simulink library "fixpt3p1_basic"  (Simulink 6.0)
settings: Solver=ode45  SolverMode=SingleTasking  StartTime=0.0  StopTime=10.0  RelTol=1e-3
undefined symbols (not defined in the file or in its folder): Bias1, Bias2, NumBits1, NumBits2, Slope1, Slope2
libraries: simulink x46, fixpt3p1_basic x2, fixpt_lib_4 x1
settings Model: CovMetricSettings=d  Creator=andyb  LastModifiedBy=andyb  ExtModeAutoUpdateStatusClock=off

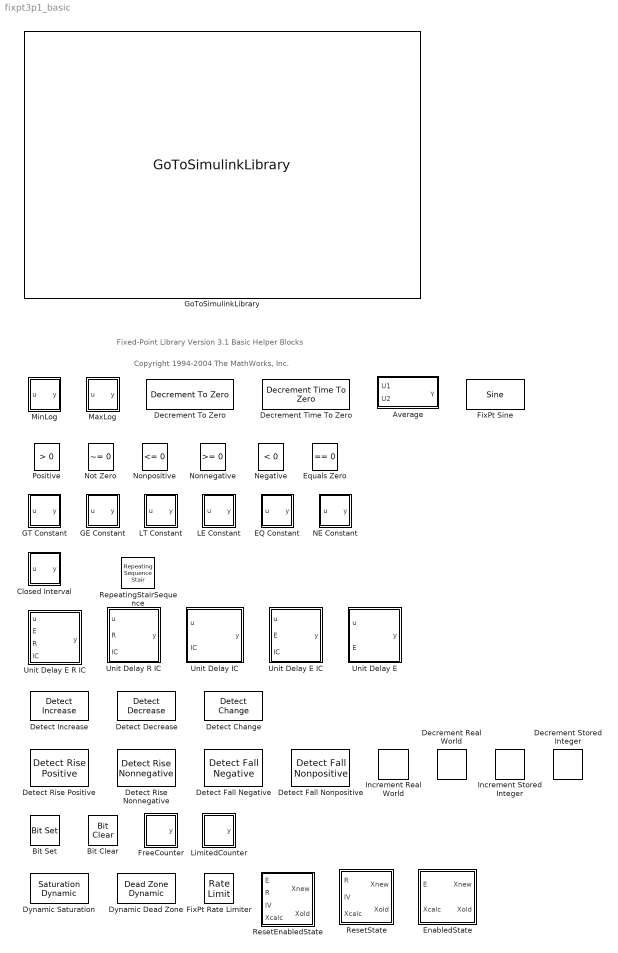
== system fixpt3p1_basic ==
  note: Fixed-Point Library Version 3.1
      | Basic Helper Blocks
  note: Copyright 1994-2004 The MathWorks, Inc.
  Average : Subsystem  PropExecContextAcrossSSBoundary=on
      mask Type: Fixed-Point Average
      mask Description: Compute the average of the two inputs.
      mask Help: fpbhelp('average');
      mask Display:
      | fprintf('(u1+u2) / 2')
      | patch([2 2 10 10 4 4 8 8 4 4 2 ],[2 10 10 8 8 6 6 4 4 2 2 ],[0 0 0],'bottom-right');
  Bit Clear : simulink/Logic and Bit Operations/Bit Clear  iBit=0
  Bit Set : simulink/Logic and Bit Operations/Bit Set  iBit=0
  Closed Interval : Subsystem  PropExecContextAcrossSSBoundary=on  mask(Fixed-Point Closed Interval){uplimit=4, lowlimit=2}
      mask prompts: uplimit "Upper limit:"; lowlimit "Lower Limit:"
      mask help: If the input is in the closed interval between the lower limit and the upper limit, then the output is TRUE, otherwise it is FALSE.
      mask Display:
      | plot([0 1],[0.3 0.3],[0.3 0.3],[0 1],[0 0.2 0.2 0.55 0.55 1],[0.35 0.35 0.6 0.6 0.35 0.35]);
      | patch([2 2 10 10 4 4 8 8 4 4 2 ],[2 10 10 8 8 6 6 4 4 2 2 ],[0 0 0],'bottom-right');
  Decrement Real World : simulink/Additional Math & Discrete/Additional Math: Increment - Decrement/Decrement Real World
  Decrement Stored Integer : simulink/Additional Math & Discrete/Additional Math: Increment - Decrement/Decrement Stored Integer
  Decrement To Zero : simulink/Additional Math & Discrete/Additional Math: Increment - Decrement/Decrement To Zero
  Decrement Time To Zero : simulink/Additional Math & Discrete/Additional Math: Increment - Decrement/Decrement Time To Zero
  Detect Change : simulink/Logic and Bit Operations/Detect Change  vinit=0
  Detect Decrease : simulink/Logic and Bit Operations/Detect Decrease  vinit=0.0
  Detect Increase : simulink/Logic and Bit Operations/Detect Increase  vinit=0.0
  Detect Fall Negative : simulink/Logic and Bit Operations/Detect Fall Negative  vinit=0
  Detect Fall Nonpositive : simulink/Logic and Bit Operations/Detect Fall Nonpositive  vinit=0
  Detect Rise Nonnegative : simulink/Logic and Bit Operations/Detect Rise Nonnegative  vinit=0
  Detect Rise Positive : simulink/Logic and Bit Operations/Detect Rise Positive  vinit=0
  Dynamic Dead Zone : simulink/Discontinuities/Dead Zone Dynamic
  Dynamic Saturation : simulink/Discontinuities/Saturation Dynamic
  EQ Constant : Subsystem  PropExecContextAcrossSSBoundary=on  mask(Fixed-Point Equal To Constant){const=3.0}
      mask prompts: const "Constant value:"
      mask help: Determine if a signal is equal to a constant.
      mask init:
      | if length(const) == 1
      |  str = ['== ',num2str(const)];
      | else
      |   str = '== C';
      | end
      mask Help: fpbhelp('eqconstant');
      mask CallbackString: fixptdialog(gcbh)
      mask Display:
      | disp(str)
      | patch([2 2 10 10 4 4 8 8 4 4 2 ],[2 10 10 8 8 6 6 4 4 2 2 ],[0 0 0],'bottom-right');
  EnabledState : Subsystem  PropExecContextAcrossSSBoundary=on
      mask Type: Fixed-Point Reset Enabled State
      mask Description:
      | Resetable Enabled State
      | Start
      |   Xold = 0.0
      | Output
      |   If E % Enabled
      |      Xnew = Xcalc
      |   else
      |      Xnew = Xold % Stays the same
      |   end
      | Update
      |     Xold = Xnew
      mask Help: fpbhelp('enabledstate');
      mask Display:
      | fprintf('State')
      | patch([2 2 10 10 4 4 8 8 4 4 2 ],[2 10 10 8 8 6 6 4 4 2 2 ],[0 0 0],'bottom-right');
  Equals Zero : simulink/Logic and Bit Operations/Compare To Zero  relop===  LogicOutDataTypeMode=uint8
  FixPt Rate Limiter : RateLimiter  RisingSlewLimit=2  FallingSlewLimit=-2
  FixPt Sine : simulink/Lookup Tables/Sine  NumDataPoints=(2^5)+1
  FreeCounter : Subsystem  PropExecContextAcrossSSBoundary=on  mask(Fixed-Point Free Counter){NumBits=16, tsamp=-1}
      mask prompts: NumBits "Number of Bits"; tsamp "Sample time:"
      mask help:
      | This block is a counter that overflows back to zero after it has reached the maximum value possible for the specified number of bits. The count is always initialized to zero.  The output is normally an unsigned integer.
      |
      | WARNING: This block is intended to overflow.  When global doubles override is on, this block will not wrap back to zero as expected.
      mask Help: fpbhelp('freecounter');
      mask Display:
      | plot( 0.05+0.9/8*[0 1 1 2 2 3 3 4 4 5 5 6 6 7 7 8 8], 0.3+0.65/3*[0 0 1 1 2 2 3 3 0 0 1 1 2 2 3 3 0] )
      | patch([2 2 10 10 4 4 8 8 4 4 2 ],[2 10 10 8 8 6 6 4 4 2 2 ],[0 0 0],'bottom-right');
  GE Constant : Subsystem  PropExecContextAcrossSSBoundary=on  mask(Fixed-Point Greater Than or Equal To Constant){const=3.0}
      mask prompts: const "Constant value:"
      mask help: Determine if a signal is greater than or equal to a constant.
      mask init:
      | if length(const) == 1
      |  str = ['>= ',num2str(const)];
      | else
      |   str = '>= C';
      | end
      mask Help: fpbhelp('geconstant');
      mask CallbackString: fixptdialog(gcbh)
      mask Display:
      | disp(str)
      | patch([2 2 10 10 4 4 8 8 4 4 2 ],[2 10 10 8 8 6 6 4 4 2 2 ],[0 0 0],'bottom-right');
  GT Constant : Subsystem  PropExecContextAcrossSSBoundary=on  mask(Fixed-Point Strictly Greater Than Constant){const=3.0}
      mask prompts: const "Constant value:"
      mask help: Determine if a signal is strictly greater than a constant.
      mask init:
      | if length(const) == 1
      |  str = ['> ',num2str(const)];
      | else
      |   str = '> C';
      | end
      mask Help: fpbhelp('gtconstant');
      mask CallbackString: fixptdialog(gcbh)
      mask Display:
      | disp(str)
      | patch([2 2 10 10 4 4 8 8 4 4 2 ],[2 10 10 8 8 6 6 4 4 2 2 ],[0 0 0],'bottom-right');
  GoToSimulinkLibrary : fixpt_lib_4/GoToSimulinkLibrary
  Increment Real World : simulink/Additional Math & Discrete/Additional Math: Increment - Decrement/Increment Real World
  Increment Stored Integer : simulink/Additional Math & Discrete/Additional Math: Increment - Decrement/Increment Stored Integer
  LE Constant : Subsystem  PropExecContextAcrossSSBoundary=on  mask(Fixed-Point Less Than Or Equal To Constant){const=3.0}
      mask prompts: const "Constant value:"
      mask help: Determine if a signal is less than or equal to a constant.
      mask init:
      | if length(const) == 1
      |  str = ['<= ',num2str(const)];
      | else
      |   str = '<= C';
      | end
      mask Help: fpbhelp('leconstant');
      mask CallbackString: fixptdialog(gcbh)
      mask Display:
      | disp(str)
      | patch([2 2 10 10 4 4 8 8 4 4 2 ],[2 10 10 8 8 6 6 4 4 2 2 ],[0 0 0],'bottom-right');
  LT Constant : Subsystem  PropExecContextAcrossSSBoundary=on  mask(Fixed-Point Strictly Less Than Constant){const=3.0}
      mask prompts: const "Constant value:"
      mask help: Determine if a signal is strictly less than a constant.
      mask init:
      | if length(const) == 1
      |  str = ['< ',num2str(const)];
      | else
      |   str = '< C';
      | end
      mask Help: fpbhelp('ltconstant');
      mask CallbackString: fixptdialog(gcbh)
      mask Display:
      | disp(str)
      | patch([2 2 10 10 4 4 8 8 4 4 2 ],[2 10 10 8 8 6 6 4 4 2 2 ],[0 0 0],'bottom-right');
  LimitedCounter : Subsystem  PropExecContextAcrossSSBoundary=on  mask(Fixed-Point Limited Counter){uplimit=7, tsamp=-1}
      mask prompts: uplimit "Upper limit:"; tsamp "Sample time:"
      mask help: This block is a counter that wraps back to zero after it has output the specified upper limit. The count is always initialized to zero. The output is normally an unsigned integer of 8, 16, or 32 bits. The smallest number of bits needed to represent the upper limit is used.
      mask init:
      | upMax = max(uplimit);
      | if upMax <= (2^8-1)
      |   nbits = 8;
      | elseif upMax <= (2^16-1)
      |   nbits = 16;
      | elseif upMax <= (2^32-1)
      |   nbits = 32;
      | elseif upMax <= (2^64-1)
      |   nbits = 64;
      | else
      |   nbits = 128;
      | end
      mask Help: fpbhelp('limitedcounter');
      mask Display:
      | plot( 0.15+0.8/8*[0 1 1 2 2 3 3 4 4 5 5 6 6 7 7 8 8], 0.3+0.65/3*[0 0 1 1 2 2 3 3 0 0 1 1 2 2 3 3 0] )
      | text(0.05,0.85,'lim')
      | patch([2 2 10 10 4 4 8 8 4 4 2 ],[2 10 10 8 8 6 6 4 4 2 2 ],[0 0 0],'bottom-right');
  MaxLog : Subsystem  PropExecContextAcrossSSBoundary=on
      mask Type: Fixed-Point Running Maximum
      mask Description:
      | Output is the maximum value of the input since the simulation began.
      | 
      | The initial value is currently set to zero!!!!!!
      mask Help: fpbhelp('maxlog');
      mask Display:
      | disp('max\nlog')
      | patch([2 2 10 10 4 4 8 8 4 4 2 ],[2 10 10 8 8 6 6 4 4 2 2 ],[0 0 0],'bottom-right');
  MinLog : Subsystem  PropExecContextAcrossSSBoundary=on
      mask Type: Fixed-Point Running Minimum
      mask Description:
      | Output is the minimum value of the input since the simulation began.
      | 
      | The initial value is currently set to zero!!!!!!
      mask Help: fpbhelp('minlog');
      mask Display:
      | disp('min\nlog')
      | patch([2 2 10 10 4 4 8 8 4 4 2 ],[2 10 10 8 8 6 6 4 4 2 2 ],[0 0 0],'bottom-right');
  NE Constant : Subsystem  PropExecContextAcrossSSBoundary=on  mask(Fixed-Point Not Equal To Constant){const=3.0}
      mask prompts: const "Constant value:"
      mask help: Determine if a signal is not equal to a constant.
      mask init:
      | if length(const) == 1
      |  str = ['~= ',num2str(const)];
      | else
      |   str = '~= C';
      | end
      mask Help: fpbhelp('neconstant');
      mask CallbackString: fixptdialog(gcbh)
      mask Display:
      | disp(str)
      | patch([2 2 10 10 4 4 8 8 4 4 2 ],[2 10 10 8 8 6 6 4 4 2 2 ],[0 0 0],'bottom-right');
  Negative : simulink/Logic and Bit Operations/Compare To Zero  relop=<  LogicOutDataTypeMode=uint8
  Nonnegative : simulink/Logic and Bit Operations/Compare To Zero  relop=>=  LogicOutDataTypeMode=uint8
  Nonpositive : simulink/Logic and Bit Operations/Compare To Zero  relop=<=  LogicOutDataTypeMode=uint8
  Not Zero : simulink/Logic and Bit Operations/Compare To Zero  relop=~=  LogicOutDataTypeMode=uint8
  Positive : simulink/Logic and Bit Operations/Compare To Zero  relop=>  LogicOutDataTypeMode=uint8
  RepeatingStairSequence : simulink/Sources/Repeating Sequence Stair  OutValues=[3 1 4 2 1].'  tsamp=-1  OutputDataTypeScalingMode=Specify via dialog  OutDataType=sfix(16)  ConRadixGroup=Best Precision: Vector-wise  OutScaling=2^-10
  ResetEnabledState : Subsystem  PropExecContextAcrossSSBoundary=on
      mask Type: Fixed-Point Reset Enabled State
      mask Description:
      | Resetable Enabled State
      | Start
      |   Xold = 0.0
      | Output
      |   If R % Reset
      |      Xnew = IV
      |   elseif E % Enabled
      |      Xnew = Xcalc
      |   else
      |      Xnew = Xold % Stays the same
      |   end
      | Update
      |     Xold = Xnew
      mask Help: fpbhelp('resetenabledstate');
      mask Display:
      | fprintf('State')
      | patch([2 2 10 10 4 4 8 8 4 4 2 ],[2 10 10 8 8 6 6 4 4 2 2 ],[0 0 0],'bottom-right');
  ResetState : Subsystem  PropExecContextAcrossSSBoundary=on
      mask Type: Fixed-Point Reset State
      mask Description:
      | Resetable State
      | Start
      |   Xold = 0.0
      | Output
      |   If R % Reset
      |      Xnew = IV
      |   else
      |      Xnew = Xcalc
      |   end
      | Update
      |     Xold = Xnew
      mask Help: fpbhelp('resetstate');
      mask Display:
      | fprintf('State')
      | patch([2 2 10 10 4 4 8 8 4 4 2 ],[2 10 10 8 8 6 6 4 4 2 2 ],[0 0 0],'bottom-right');
  Unit Delay E : Subsystem  PropExecContextAcrossSSBoundary=on  mask(Fixed-Point Unit Delay Enable){vinit=0.0, tsamp=-1}
      mask prompts: vinit "Initial condition:"; tsamp "Sample time:"
      mask help:
      | Enabled Unit Delay
      | Start
      |   x = IC   % Initial Condition
      | Output
      |   y = IC   % Initial Condition
      | Update
      |   If E   % Enabled
      |      x = u
      |   else
      |      % x stays the same
      |   end
      mask Help: fpbhelp('unitdelaye');
      mask Display:
      | dpoly(1,[1 0],'z')
      | patch([2 2 10 10 4 4 8 8 4 4 2 ],[2 10 10 8 8 6 6 4 4 2 2 ],[0 0 0],'bottom-right');
  Unit Delay E IC : Subsystem  PropExecContextAcrossSSBoundary=on  mask(Fixed-Point Unit Delay Enable Initial_Condition){tsamp=-1}
      mask prompts: tsamp "Sample time:"
      mask help:
      | Enabled Unit Delay with External Initial Condition
      | Start
      |   x = IC   % Initial Condition
      | Output
      |   y = IC   % Initial Condition
      | Update
      |   If E   % Enabled
      |      x = u
      |   else
      |      % x stays the same
      |   end
      mask Help: fpbhelp('unitdelayeic');
      mask Display:
      | dpoly(1,[1 0],'z')
      | patch([2 2 10 10 4 4 8 8 4 4 2 ],[2 10 10 8 8 6 6 4 4 2 2 ],[0 0 0],'bottom-right');
  Unit Delay E R IC : Subsystem  PropExecContextAcrossSSBoundary=on  mask(Fixed-Point Unit Delay Reset Enable Initial_Condition){tsamp=-1}
      mask prompts: tsamp "Sample time:"
      mask help:
      | Resetable Enabled Unit Delay with External Initial Condition
      | Start
      |   x = IC   % Initial Condition
      | Output
      |   If R   % Reset
      |      y = IC   % Initial Condition
      |   else
      |      y = x
      |   end
      | Update
      |   If R   % Reset
      |      x = IC   % Initial Condition
      |   elseif E   % Enabled
      |      x = u
      |   else
      |      % x stays the same
      |   end
      mask Help: fpbhelp('unitdelayeric');
      mask Display:
      | dpoly(1,[1 0],'z')
      | patch([2 2 10 10 4 4 8 8 4 4 2 ],[2 10 10 8 8 6 6 4 4 2 2 ],[0 0 0],'bottom-right');
  Unit Delay IC : Subsystem  PropExecContextAcrossSSBoundary=on  mask(Fixed-Point Unit Delay Initial_Condition){tsamp=-1}
      mask prompts: tsamp "Sample time:"
      mask help:
      | Unit Delay with External Initial Condition
      | Start
      |   x = IC   % Initial Condition
      | Output
      |   y = x
      | Update
      |   x = u
      mask Help: fpbhelp('unitdelayic');
      mask Display:
      | dpoly(1,[1 0],'z')
      | patch([2 2 10 10 4 4 8 8 4 4 2 ],[2 10 10 8 8 6 6 4 4 2 2 ],[0 0 0],'bottom-right');
  Unit Delay R IC : Subsystem  PropExecContextAcrossSSBoundary=on  mask(Fixed-Point Unit Delay Reset Initial_Condition){tsamp=-1}
      mask prompts: tsamp "Sample time:"
      mask help:
      | Resetable Unit Delay with External Initial Condition
      | Start
      |   x = IC   % Initial Condition
      | Output
      |   If R   % Reset
      |      y = IC   % Initial Condition
      |   else
      |      y = x
      |   end
      | Update
      |   If R   % Reset
      |      x = IC   % Initial Condition
      |   else
      |      x = u
      |   end
      mask Help: fpbhelp('unitdelayric');
      mask Display:
      | dpoly(1,[1 0],'z')
      | patch([2 2 10 10 4 4 8 8 4 4 2 ],[2 10 10 8 8 6 6 4 4 2 2 ],[0 0 0],'bottom-right');

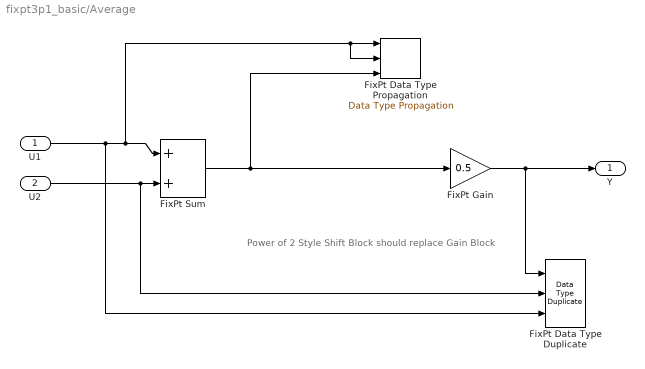
== system fixpt3p1_basic/Average ==
  note: Power of 2 Style Shift Block
      | should replace Gain Block
  U1 : Inport  LatchInput=off
  U2 : Inport  Port=2  LatchInput=off
  FixPt Data Type Duplicate : simulink/Signal Attributes/Data Type Duplicate  NumInputPorts=3
  FixPt Data Type Propagation : simulink/Signal Attributes/Data Type Propagation  PropDataType=sfix(16)  IfRefDouble=double  IfRefSingle=single  IsSigned=IsSigned1  NumBitsBase=NumBits1  NumBitsMult=2  NumBitsAdd=0  NumBitsAllowFinal=1:128  PropScaling=2^-10  ValuesUsedBestPrec=[5 -7]  SlopeBase=Slope1  SlopeMult=1  SlopeAdd=0  BiasBase=Bias1+Bias2  BiasMult=1  BiasAdd=0
  FixPt Gain : Gain  Gain=0.5  ParameterDataTypeMode=Specify via dialog  ParameterDataType=ufix(8)  ParameterScalingMode=Use specified scaling  ParameterScaling=2^-1  OutScaling=2^-10
  FixPt Sum : Sum  OutScaling=2^-10
  Y : Outport  InitialOutput=0
  wires:
  FixPt Gain/1 -> Y/1, FixPt Data Type Duplicate/1
  U1/1 -> FixPt Sum/1, FixPt Data Type Propagation/1, FixPt Data Type Propagation/2, FixPt Data Type Duplicate/3
  U2/1 -> FixPt Sum/2, FixPt Data Type Duplicate/2
  FixPt Sum/1 -> FixPt Gain/1, FixPt Data Type Propagation/3

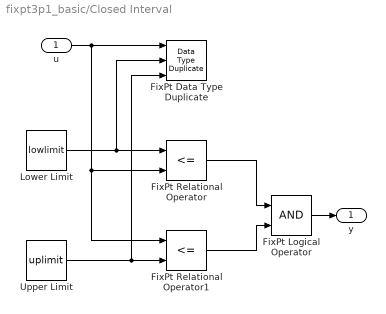
== system fixpt3p1_basic/Closed Interval ==
  u : Inport  LatchInput=off
  FixPt Data Type Duplicate : simulink/Signal Attributes/Data Type Duplicate  NumInputPorts=3
  FixPt Logical Operator : Logic  AllPortsSameDT=off  OutDataTypeMode=Specify via dialog
  FixPt Relational Operator : RelationalOperator  Operator=<=  LogicOutDataTypeMode=Specify via dialog  ZeroCross=off
  FixPt Relational Operator1 : RelationalOperator  Operator=<=  LogicOutDataTypeMode=Specify via dialog  ZeroCross=off
  Lower Limit : Constant  Value=lowlimit  ConRadixGroup=Best Precision: Vector-wise  OutScaling=2^-1000
  Upper Limit : Constant  Value=uplimit  ConRadixGroup=Best Precision: Vector-wise  OutScaling=2^-1000
  y : Outport
  wires:
  Lower Limit/1 -> FixPt Relational Operator/1, FixPt Data Type Duplicate/2
  Upper Limit/1 -> FixPt Relational Operator1/2, FixPt Data Type Duplicate/3
  FixPt Relational Operator/1 -> FixPt Logical Operator/1
  FixPt Relational Operator1/1 -> FixPt Logical Operator/2
  u/1 -> FixPt Data Type Duplicate/1, FixPt Relational Operator/2, FixPt Relational Operator1/1
  FixPt Logical Operator/1 -> y/1

== system fixpt3p1_basic/EQ Constant ==
  u : Inport  LatchInput=off
  FixPt Constant : Constant  Value=const  OutScaling=1
  FixPt Data Type Duplicate : simulink/Signal Attributes/Data Type Duplicate  NumInputPorts=2
  FixPt Relational Operator : RelationalOperator  Operator===  LogicOutDataTypeMode=Specify via dialog  ZeroCross=off
  y : Outport
  wires:
  FixPt Relational Operator/1 -> y/1
  FixPt Constant/1 -> FixPt Data Type Duplicate/2, FixPt Relational Operator/2
  u/1 -> FixPt Data Type Duplicate/1, FixPt Relational Operator/1

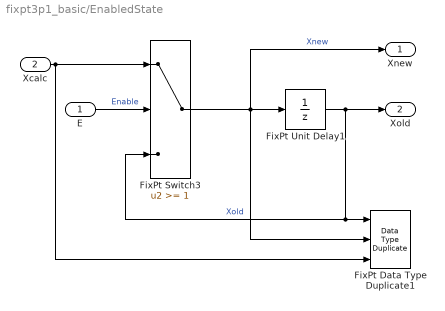
== system fixpt3p1_basic/EnabledState ==
  E : Inport  LatchInput=off
  Xcalc : Inport  Port=2  LatchInput=off
  FixPt Data Type Duplicate1 : simulink/Signal Attributes/Data Type Duplicate  NumInputPorts=3
  FixPt Switch3 : Switch  Threshold=1  ZeroCross=off
  FixPt Unit Delay1 : UnitDelay  X0=0.0  SampleTime=-1
  Xnew : Outport
  Xold : Outport  Port=2
  wires:
  E/1 -> FixPt Switch3/2  "Enable"
  Xcalc/1 -> FixPt Data Type Duplicate1/3, FixPt Switch3/1
  FixPt Switch3/1 -> Xnew/1, FixPt Data Type Duplicate1/2, FixPt Unit Delay1/1  "Xnew"
  FixPt Unit Delay1/1 -> Xold/1, FixPt Switch3/3, FixPt Data Type Duplicate1/1  "Xold"

== system fixpt3p1_basic/FreeCounter ==
  FixPt Data Type Propagation : simulink/Signal Attributes/Data Type Propagation  PropDataTypeMode=Specify via dialog  PropDataType=uint(NumBits)  IfRefDouble=double  IfRefSingle=single  IsSigned=IsSigned1 or IsSigned2  NumBitsBase=max([NumBits1 NumBits2])  NumBitsMult=1  NumBitsAdd=0  NumBitsAllowFinal=1:128  PropScalingMode=Specify via dialog  PropScaling=1  ValuesUsedBestPrec=[5 -7]  SlopeBase=min([Slope1 Slope2])  SlopeMult=1  SlopeAdd=0  BiasBase=Bias1  BiasMult=1  BiasAdd=0
  FixPt Unit Delay2 : UnitDelay  X0=0.0  SampleTime=tsamp
  Increment Real World : fixpt3p1_basic/Increment Real World
  y : Outport
  wires:
  Increment Real World/1 -> FixPt Unit Delay2/1, FixPt Data Type Propagation/1, FixPt Data Type Propagation/3, FixPt Data Type Propagation/2
  FixPt Unit Delay2/1 -> y/1, Increment Real World/1

== system fixpt3p1_basic/GE Constant ==
  u : Inport  LatchInput=off
  FixPt Constant : Constant  Value=const  OutScaling=1
  FixPt Data Type Duplicate : simulink/Signal Attributes/Data Type Duplicate  NumInputPorts=2
  FixPt Relational Operator : RelationalOperator  LogicOutDataTypeMode=Specify via dialog  ZeroCross=off
  y : Outport
  wires:
  u/1 -> FixPt Relational Operator/1, FixPt Data Type Duplicate/1
  FixPt Constant/1 -> FixPt Relational Operator/2, FixPt Data Type Duplicate/2
  FixPt Relational Operator/1 -> y/1

== system fixpt3p1_basic/GT Constant ==
  u : Inport  LatchInput=off
  FixPt Constant : Constant  Value=const  OutScaling=1
  FixPt Data Type Duplicate : simulink/Signal Attributes/Data Type Duplicate  NumInputPorts=2
  FixPt Relational Operator : RelationalOperator  Operator=>  LogicOutDataTypeMode=Specify via dialog  ZeroCross=off
  y : Outport
  wires:
  FixPt Relational Operator/1 -> y/1
  FixPt Constant/1 -> FixPt Data Type Duplicate/2, FixPt Relational Operator/2
  u/1 -> FixPt Data Type Duplicate/1, FixPt Relational Operator/1

== system fixpt3p1_basic/LE Constant ==
  u : Inport  LatchInput=off
  FixPt Constant : Constant  Value=const  OutScaling=1
  FixPt Data Type Duplicate : simulink/Signal Attributes/Data Type Duplicate  NumInputPorts=2
  FixPt Relational Operator : RelationalOperator  Operator=<=  LogicOutDataTypeMode=Specify via dialog  ZeroCross=off
  y : Outport
  wires:
  u/1 -> FixPt Relational Operator/1, FixPt Data Type Duplicate/1
  FixPt Constant/1 -> FixPt Relational Operator/2, FixPt Data Type Duplicate/2
  FixPt Relational Operator/1 -> y/1

== system fixpt3p1_basic/LT Constant ==
  u : Inport  LatchInput=off
  FixPt Constant : Constant  Value=const  OutScaling=1
  FixPt Data Type Duplicate : simulink/Signal Attributes/Data Type Duplicate  NumInputPorts=2
  FixPt Relational Operator : RelationalOperator  Operator=<  LogicOutDataTypeMode=Specify via dialog  ZeroCross=off
  y : Outport
  wires:
  FixPt Relational Operator/1 -> y/1
  FixPt Constant/1 -> FixPt Data Type Duplicate/2, FixPt Relational Operator/2
  u/1 -> FixPt Data Type Duplicate/1, FixPt Relational Operator/1

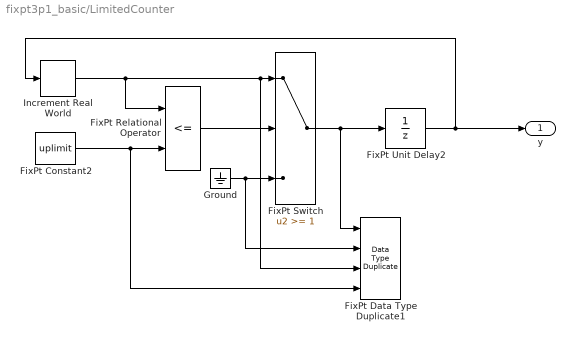
== system fixpt3p1_basic/LimitedCounter ==
  FixPt Constant2 : Constant  Value=uplimit  OutDataTypeMode=Specify via dialog  OutDataType=uint(nbits)  OutScaling=1
  FixPt Data Type Duplicate1 : simulink/Signal Attributes/Data Type Duplicate  NumInputPorts=4
  FixPt Relational Operator : RelationalOperator  Operator=<=  LogicOutDataTypeMode=Specify via dialog  ZeroCross=off
  FixPt Switch : Switch  Threshold=1  ZeroCross=off
  FixPt Unit Delay2 : UnitDelay  X0=0.0  SampleTime=tsamp
  Ground : Ground
  Increment Real World : fixpt3p1_basic/Increment Real World
  y : Outport
  wires:
  FixPt Constant2/1 -> FixPt Data Type Duplicate1/4, FixPt Relational Operator/2
  FixPt Relational Operator/1 -> FixPt Switch/2
  FixPt Unit Delay2/1 -> Increment Real World/1, y/1
  FixPt Switch/1 -> FixPt Unit Delay2/1, FixPt Data Type Duplicate1/1
  Increment Real World/1 -> FixPt Data Type Duplicate1/3, FixPt Switch/1, FixPt Relational Operator/1
  Ground/1 -> FixPt Switch/3, FixPt Data Type Duplicate1/2

== system fixpt3p1_basic/MaxLog ==
  u : Inport  LatchInput=off
  FixPt Data Type Duplicate : simulink/Signal Attributes/Data Type Duplicate  NumInputPorts=3
  FixPt Unit Delay : UnitDelay  X0=0.0  SampleTime=-1
  max low : MinMax  Function=max  Inputs=2  OutScaling=2^-10  ZeroCross=off
  y : Outport
  wires:
  max low/1 -> FixPt Data Type Duplicate/1, FixPt Unit Delay/1
  u/1 -> FixPt Data Type Duplicate/3, max low/1
  FixPt Unit Delay/1 -> FixPt Data Type Duplicate/2, max low/2, y/1

== system fixpt3p1_basic/MinLog ==
  u : Inport  LatchInput=off
  FixPt Data Type Duplicate : simulink/Signal Attributes/Data Type Duplicate  NumInputPorts=3
  FixPt Unit Delay : UnitDelay  X0=0.0  SampleTime=-1
  min : MinMax  Inputs=2  OutScaling=2^-10  ZeroCross=off
  y : Outport
  wires:
  FixPt Unit Delay/1 -> min/2, FixPt Data Type Duplicate/2, y/1
  u/1 -> min/1, FixPt Data Type Duplicate/3
  min/1 -> FixPt Unit Delay/1, FixPt Data Type Duplicate/1

== system fixpt3p1_basic/NE Constant ==
  u : Inport  LatchInput=off
  FixPt Constant : Constant  Value=const  OutScaling=1
  FixPt Data Type Duplicate : simulink/Signal Attributes/Data Type Duplicate  NumInputPorts=2
  FixPt Relational Operator : RelationalOperator  Operator=~=  LogicOutDataTypeMode=Specify via dialog  ZeroCross=off
  y : Outport
  wires:
  u/1 -> FixPt Relational Operator/1, FixPt Data Type Duplicate/1
  FixPt Constant/1 -> FixPt Relational Operator/2, FixPt Data Type Duplicate/2
  FixPt Relational Operator/1 -> y/1

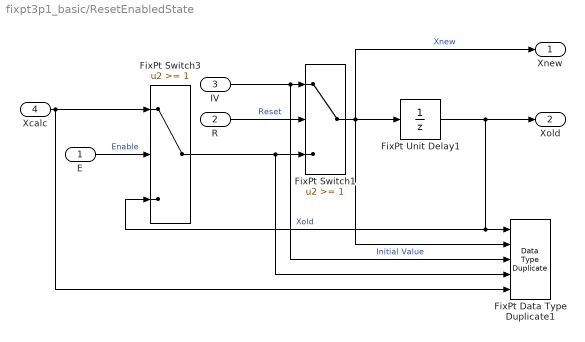
== system fixpt3p1_basic/ResetEnabledState ==
  E : Inport  LatchInput=off
  R : Inport  Port=2  LatchInput=off
  IV : Inport  Port=3  LatchInput=off
  Xcalc : Inport  Port=4  LatchInput=off
  FixPt Data Type Duplicate1 : simulink/Signal Attributes/Data Type Duplicate  NumInputPorts=5
  FixPt Switch1 : Switch  Threshold=1  ZeroCross=off
  FixPt Switch3 : Switch  Threshold=1  ZeroCross=off
  FixPt Unit Delay1 : UnitDelay  X0=0.0  SampleTime=-1
  Xnew : Outport
  Xold : Outport  Port=2
  wires:
  R/1 -> FixPt Switch1/2  "Reset"
  FixPt Switch1/1 -> FixPt Unit Delay1/1, FixPt Data Type Duplicate1/2, Xnew/1  "Xnew"
  FixPt Unit Delay1/1 -> FixPt Data Type Duplicate1/1, FixPt Switch3/3, Xold/1  "Xold"
  FixPt Switch3/1 -> FixPt Switch1/3, FixPt Data Type Duplicate1/4
  Xcalc/1 -> FixPt Switch3/1, FixPt Data Type Duplicate1/5
  IV/1 -> FixPt Switch1/1, FixPt Data Type Duplicate1/3  "Initial Value"
  E/1 -> FixPt Switch3/2  "Enable"

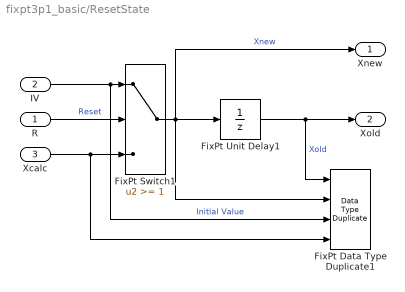
== system fixpt3p1_basic/ResetState ==
  R : Inport  LatchInput=off
  IV : Inport  Port=2  LatchInput=off
  Xcalc : Inport  Port=3  LatchInput=off
  FixPt Data Type Duplicate1 : simulink/Signal Attributes/Data Type Duplicate  NumInputPorts=4
  FixPt Switch1 : Switch  Threshold=1  ZeroCross=off
  FixPt Unit Delay1 : UnitDelay  X0=0.0  SampleTime=-1
  Xnew : Outport
  Xold : Outport  Port=2
  wires:
  IV/1 -> FixPt Data Type Duplicate1/3, FixPt Switch1/1  "Initial Value"
  Xcalc/1 -> FixPt Data Type Duplicate1/4, FixPt Switch1/3
  FixPt Unit Delay1/1 -> Xold/1, FixPt Data Type Duplicate1/1  "Xold"
  FixPt Switch1/1 -> Xnew/1, FixPt Data Type Duplicate1/2, FixPt Unit Delay1/1  "Xnew"
  R/1 -> FixPt Switch1/2  "Reset"

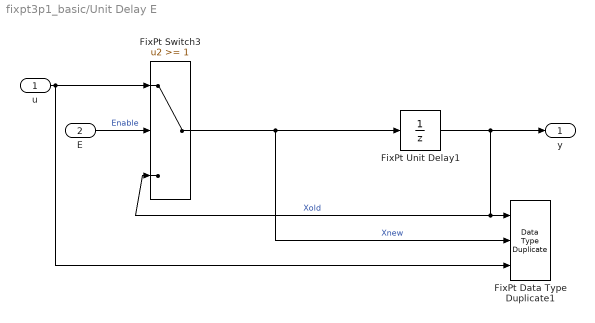
== system fixpt3p1_basic/Unit Delay E ==
  u : Inport  LatchInput=off
  E : Inport  Port=2  LatchInput=off
  FixPt Data Type Duplicate1 : simulink/Signal Attributes/Data Type Duplicate  NumInputPorts=3
  FixPt Switch3 : Switch  Threshold=1  ZeroCross=off
  FixPt Unit Delay1 : UnitDelay  X0=vinit  SampleTime=tsamp
  y : Outport
  wires:
  FixPt Unit Delay1/1 -> FixPt Data Type Duplicate1/1, FixPt Switch3/3, y/1  "Xold"
  FixPt Switch3/1 -> FixPt Data Type Duplicate1/2, FixPt Unit Delay1/1  "Xnew"
  u/1 -> FixPt Switch3/1, FixPt Data Type Duplicate1/3
  E/1 -> FixPt Switch3/2  "Enable"

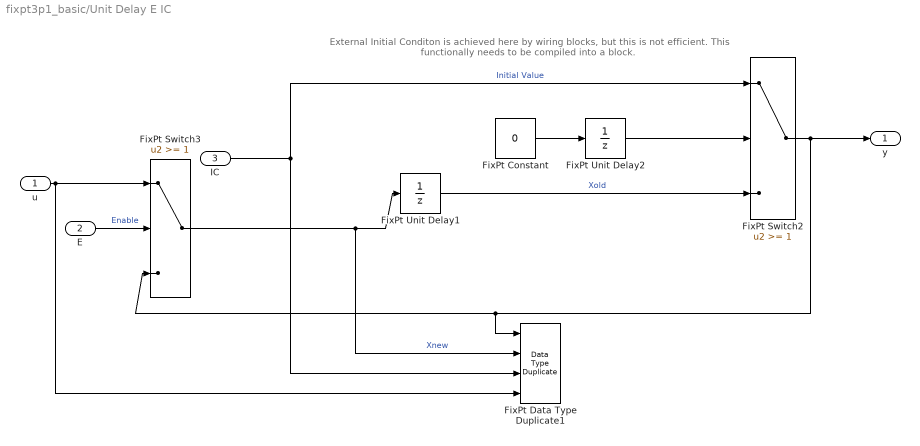
== system fixpt3p1_basic/Unit Delay E IC ==
  note: External Initial Conditon is achieved here by wiring blocks,
      | but this is not efficient.  This functionally needs to
      | be compiled into a block.
  u : Inport  LatchInput=off
  E : Inport  Port=2  LatchInput=off
  IC : Inport  Port=3  LatchInput=off
  FixPt Constant : Constant  Value=0  OutDataTypeMode=Specify via dialog  OutDataType=uint(8)  OutScaling=1
  FixPt Data Type Duplicate1 : simulink/Signal Attributes/Data Type Duplicate  NumInputPorts=4
  FixPt Switch2 : Switch  Threshold=1  ZeroCross=off
  FixPt Switch3 : Switch  Threshold=1  ZeroCross=off
  FixPt Unit Delay1 : UnitDelay  X0=0.0  SampleTime=tsamp
  FixPt Unit Delay2 : UnitDelay  X0=1  SampleTime=tsamp
  y : Outport
  wires:
  FixPt Unit Delay1/1 -> FixPt Switch2/3  "Xold"
  FixPt Switch2/1 -> FixPt Data Type Duplicate1/1, FixPt Switch3/3, y/1
  FixPt Unit Delay2/1 -> FixPt Switch2/2
  FixPt Constant/1 -> FixPt Unit Delay2/1
  FixPt Switch3/1 -> FixPt Unit Delay1/1, FixPt Data Type Duplicate1/2  "Xnew"
  u/1 -> FixPt Switch3/1, FixPt Data Type Duplicate1/4
  IC/1 -> FixPt Data Type Duplicate1/3, FixPt Switch2/1  "Initial Value"
  E/1 -> FixPt Switch3/2  "Enable"

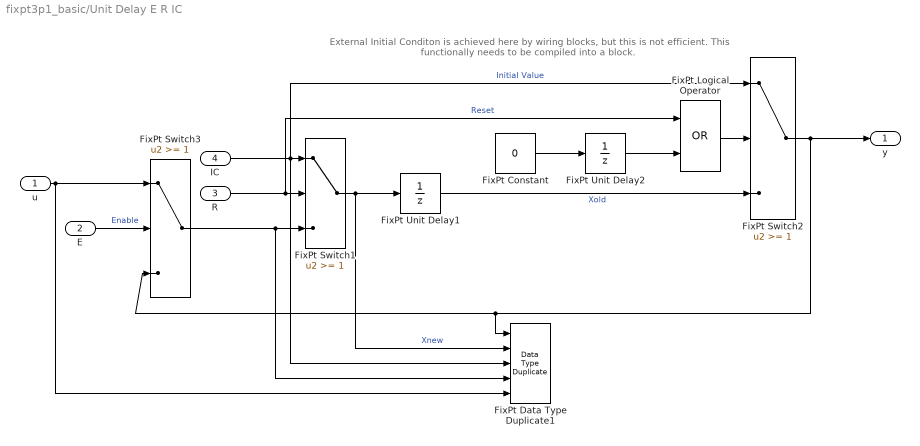
== system fixpt3p1_basic/Unit Delay E R IC ==
  note: External Initial Conditon is achieved here by wiring blocks,
      | but this is not efficient.  This functionally needs to
      | be compiled into a block.
  u : Inport  LatchInput=off
  E : Inport  Port=2  LatchInput=off
  R : Inport  Port=3  LatchInput=off
  IC : Inport  Port=4  LatchInput=off
  FixPt Constant : Constant  Value=0  OutDataTypeMode=Specify via dialog  OutDataType=uint(8)  OutScaling=1
  FixPt Data Type Duplicate1 : simulink/Signal Attributes/Data Type Duplicate  NumInputPorts=5
  FixPt Logical Operator : Logic  Operator=OR  AllPortsSameDT=off  OutDataTypeMode=Specify via dialog
  FixPt Switch1 : Switch  Threshold=1  ZeroCross=off
  FixPt Switch2 : Switch  Threshold=1  ZeroCross=off
  FixPt Switch3 : Switch  Threshold=1  ZeroCross=off
  FixPt Unit Delay1 : UnitDelay  X0=0.0  SampleTime=tsamp
  FixPt Unit Delay2 : UnitDelay  X0=1  SampleTime=tsamp
  y : Outport
  wires:
  E/1 -> FixPt Switch3/2  "Enable"
  IC/1 -> FixPt Switch1/1, FixPt Switch2/1, FixPt Data Type Duplicate1/3  "Initial Value"
  u/1 -> FixPt Data Type Duplicate1/5, FixPt Switch3/1
  FixPt Switch3/1 -> FixPt Data Type Duplicate1/4, FixPt Switch1/3
  FixPt Switch1/1 -> FixPt Data Type Duplicate1/2, FixPt Unit Delay1/1  "Xnew"
  R/1 -> FixPt Switch1/2, FixPt Logical Operator/1  "Reset"
  FixPt Constant/1 -> FixPt Unit Delay2/1
  FixPt Unit Delay2/1 -> FixPt Logical Operator/2
  FixPt Switch2/1 -> y/1, FixPt Switch3/3, FixPt Data Type Duplicate1/1
  FixPt Unit Delay1/1 -> FixPt Switch2/3  "Xold"
  FixPt Logical Operator/1 -> FixPt Switch2/2

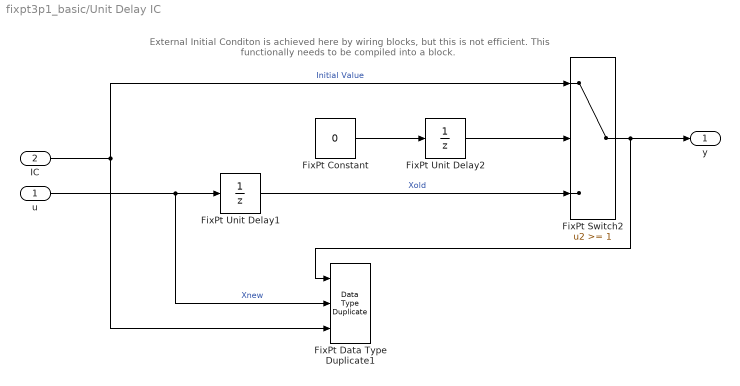
== system fixpt3p1_basic/Unit Delay IC ==
  note: External Initial Conditon is achieved here by wiring blocks,
      | but this is not efficient.  This functionally needs to
      | be compiled into a block.
  u : Inport  LatchInput=off
  IC : Inport  Port=2  LatchInput=off
  FixPt Constant : Constant  Value=0  OutDataTypeMode=Specify via dialog  OutDataType=uint(8)  OutScaling=1
  FixPt Data Type Duplicate1 : simulink/Signal Attributes/Data Type Duplicate  NumInputPorts=3
  FixPt Switch2 : Switch  Threshold=1  ZeroCross=off
  FixPt Unit Delay1 : UnitDelay  X0=0.0  SampleTime=tsamp
  FixPt Unit Delay2 : UnitDelay  X0=1  SampleTime=tsamp
  y : Outport
  wires:
  IC/1 -> FixPt Data Type Duplicate1/3, FixPt Switch2/1  "Initial Value"
  u/1 -> FixPt Data Type Duplicate1/2, FixPt Unit Delay1/1  "Xnew"
  FixPt Constant/1 -> FixPt Unit Delay2/1
  FixPt Unit Delay2/1 -> FixPt Switch2/2
  FixPt Switch2/1 -> FixPt Data Type Duplicate1/1, y/1
  FixPt Unit Delay1/1 -> FixPt Switch2/3  "Xold"

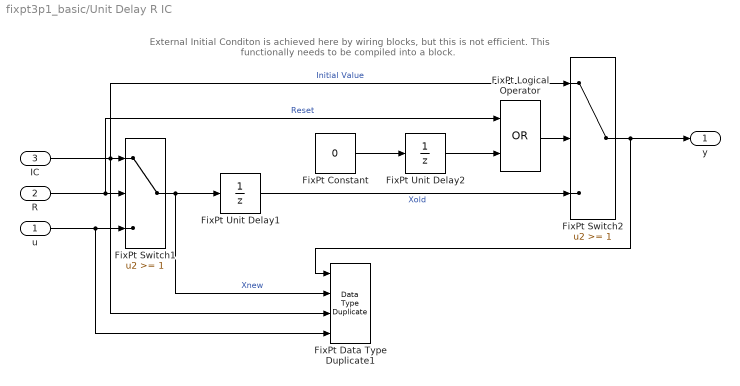
== system fixpt3p1_basic/Unit Delay R IC ==
  note: External Initial Conditon is achieved here by wiring blocks,
      | but this is not efficient.  This functionally needs to
      | be compiled into a block.
  u : Inport  LatchInput=off
  R : Inport  Port=2  LatchInput=off
  IC : Inport  Port=3  LatchInput=off
  FixPt Constant : Constant  Value=0  OutDataTypeMode=Specify via dialog  OutDataType=uint(8)  OutScaling=1
  FixPt Data Type Duplicate1 : simulink/Signal Attributes/Data Type Duplicate  NumInputPorts=4
  FixPt Logical Operator : Logic  Operator=OR  AllPortsSameDT=off  OutDataTypeMode=Specify via dialog
  FixPt Switch1 : Switch  Threshold=1  ZeroCross=off
  FixPt Switch2 : Switch  Threshold=1  ZeroCross=off
  FixPt Unit Delay1 : UnitDelay  X0=0.0  SampleTime=tsamp
  FixPt Unit Delay2 : UnitDelay  X0=1  SampleTime=tsamp
  y : Outport
  wires:
  FixPt Logical Operator/1 -> FixPt Switch2/2
  FixPt Unit Delay1/1 -> FixPt Switch2/3  "Xold"
  FixPt Switch2/1 -> y/1, FixPt Data Type Duplicate1/1
  FixPt Unit Delay2/1 -> FixPt Logical Operator/2
  FixPt Constant/1 -> FixPt Unit Delay2/1
  R/1 -> FixPt Logical Operator/1, FixPt Switch1/2  "Reset"
  FixPt Switch1/1 -> FixPt Unit Delay1/1, FixPt Data Type Duplicate1/2  "Xnew"
  u/1 -> FixPt Switch1/3, FixPt Data Type Duplicate1/4
  IC/1 -> FixPt Data Type Duplicate1/3, FixPt Switch2/1, FixPt Switch1/1  "Initial Value"
